simulink model "CostasLoop"  (R2025a)
settings: Solver=ode45  StartTime=0.0  StopTime=5000  RelTol=1e-3  EnableMultiTasking=on
PreLoadFcn:
  | CostasLoop_PreLoadFcn
undefined symbols (not defined in the file): h, k_i, k_p, S, vsva2197, xcvc1902
libraries: hdlBasic x33, dspmlti4 x2, hdlUtilities x1, vmcUtilities x1
settings Model: ExtModeTrigMode=oneshot  ExtModeArmWhenConnect=off  Creator=alexc  LastModifiedBy=robg
settings SolverCC: AlgebraicLoopSolver=TrustRegion
settings DataIOCC: SaveFormat=Array  SignalLoggingSaveFormat=ModelDataLogs  ReturnWorkspaceOutputs=off  SignalLoggingName=sigsOut
settings OptimizationCC: BlockReduction=off  BooleanDataType=off  DefaultParameterBehavior=Inlined  ExpressionDepthLimit=2147483647.0  InitFltsAndDblsToZero=on  LifeSpan=inf
settings DebuggingCC: SaveWithParameterizedLinksMsg=none  UnderspecifiedInitializationDetection=Classic  MergeDetectMultiDrivingBlocksExec=none  SignalResolutionControl=TryResolveAllWithWarning  MultiTaskDSMMsg=warning  MultiTaskCondExecSysMsg=none  FcnCallInpInsideContextMsg=warning  UnconnectedInputMsg=warning  UnconnectedOutputMsg=warning  UnconnectedLineMsg=warning  StateNameClashWarn=warning  SFUnexpectedBacktrackingDiag=warning  SFNoUnconditionalDefaultTransitionDiag=warning  SFExecutionAtInitializationDiag=none  ArithmeticOperatorsInVariantConditions=warning
settings HardwareCC: ProdBitPerPointer=32.0  ProdBitPerSizeT=32.0  ProdBitPerPtrDiffT=32.0  ProdLargestAtomicFloat=None  ProdIntDivRoundTo=Undefined  ProdEndianess=Unspecified  ProdWordSize=32.0  ProdHWDeviceType=32-bit Generic  TargetUnknown=on
settings ModelReferenceCC: EnableRefExpFcnMdlSchedulingChecks=on  PropagateSignalLabelsOutOfModel=off
settings SFSimCC: SimUseLocalCustomCode=off  CustomCodeUndefinedFunction=UseInterfaceOnly
settings RTWCC: RTWUseLocalCustomCode=off  GPUComputeCapability=3.5  DLArmComputeVersion=19.05
settings CodeAppCC: StateflowObjectComments=on
settings GRTTargetCC: TargetFcnLib=ansi_tfl_tmw.mat  TargetLangStandard=C89/C90 (ANSI)  CombineOutputUpdateFcns=off  GRTInterface=on
settings ConfigComp: CovMetricSettings=dw  CovSaveCumulativeToWorkspaceVar=on  CovSaveSingleToWorkspaceVar=on  CovExternalEMLEnable=off

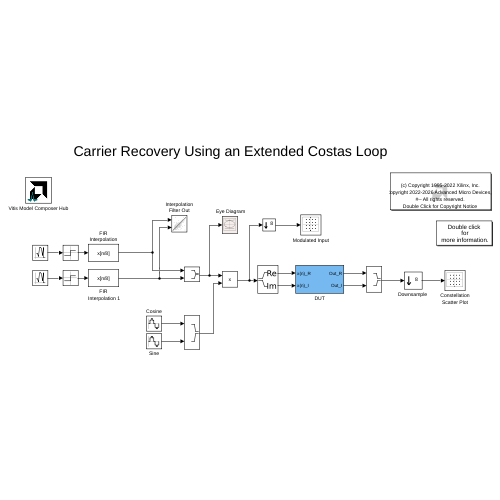
[thumbnail: Simulink's stored preview of the top-level diagram]
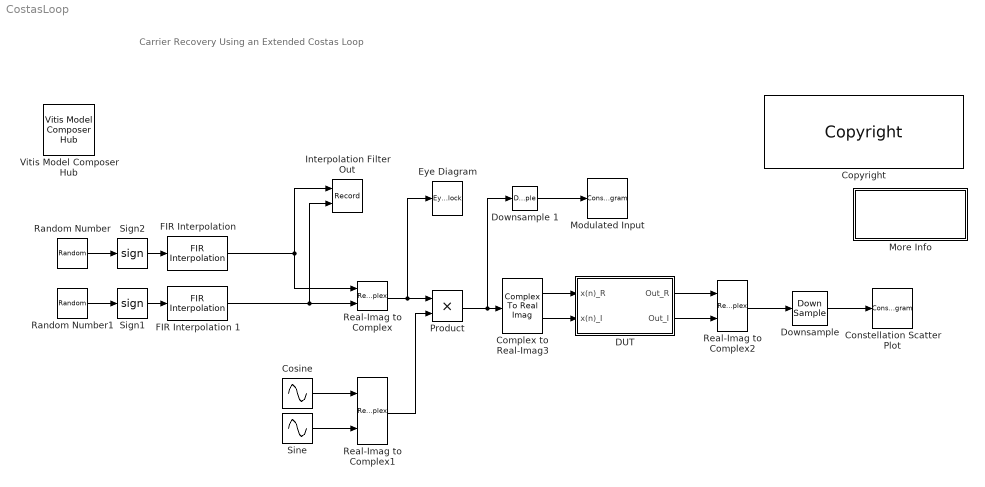
== system CostasLoop ==
  note: Carrier Recovery Using an Extended Costas Loop
  " Eye Diagram" : EyeDiagramBlock  Tag=EyeDiagram  WindowPosition=[560.000000,350.000000,800.000000,500.000000,]  Visible=on  ScopeFrameLocation=window  SamplesPerSymbol=32  SampleOffset=16  SymbolsPerTrace=1  Title=Eye Diagram  YLimits=[-2.0252 2.0024]  ColorFading=on
  Complex to Real-Imag3 : ComplexToRealImag
  Constellation Scatter Plot : ConstellationDiagram  Tag=ScatterPlot  WindowPosition=[1252.000000,116.000000,568.000000,545.000000,]  Visible=on  ScopeFrameLocation=window  SamplesPerSymbol=4  SymbolsToDisplaySource=Property  SymbolsToDisplay=40  Title=Scatter Plot  AxesLimits=[-1.5 1.5]  ColorFading=on  DefaultConfigurationName=comm.scopes.ConstellationDiagramBlockCfg
  Copyright : hdlUtilities/Copyright  copyrighttext="(c) Copyright 1995-2022 Xilinx, Inc. <br>(c) Copyright 2022-2026 Advanced Micro Devices, Inc. All rights reserved.<br><br>This document  contains proprietary, confidential information that may be used, copied and/or disclosed only as authorized by a valid licensing agreement with Advanced Micro Devices, Inc. This copyright notice must be retained on all authorized copies.<br><br> This code is provided \"as is\". Advanced Micro Devices, Inc. makes, and the end user receives, no warranties or conditions, express, implied, statutory or otherwise, and Advanced Micro Devices, Inc. specifically disclaims any implied warranties of merchantability, <br>non-infringement, or fitness for a particular purpose."  block_type=copyright
  Cosine : Sin  Frequency=2*pi*0.001/8  Phase=pi/2  SampleTime=8
  DUT : Subsystem
  "Downsample " : DownSample  N=8  InputProcessing=Inherited (this choice will be removed - see release notes)  RateOptions=Allow multirate processing
  Downsample 1 : DownSample  N=8  phase=2  InputProcessing=Inherited (this choice will be removed - see release notes)  RateOptions=Allow multirate processing
  "FIR Interpolation " : dspmlti4/FIR Interpolation  FilterSource=Dialog parameters  PrivateCoeffs=0  h=[h]  L=8  FilterObject=Hm_firinterp  InputProcessing=Columns as channels (frame based)  framing=Allow multirate processing  outputBufInitCond=0  roundingMode=Floor  overflowMode=off  firstCoeffDataTypeStr=Inherit: Same word length as input  firstCoeffMin=[]  firstCoeffMax=[]  firstCoeffLastDataTypeStr=Inherit: Same word length as input  outputDataTypeStr=Inherit: Same as accumulator  outputMin=[]  outputMax=[]  outputLastDataTypeStr=Inherit: Same as accumulator
  FIR Interpolation 1 : dspmlti4/FIR Interpolation  FilterSource=Dialog parameters  PrivateCoeffs=0  h=[h]  L=8  FilterObject=Hm_firinterp  InputProcessing=Columns as channels (frame based)  framing=Allow multirate processing  outputBufInitCond=0  roundingMode=Floor  overflowMode=off  firstCoeffDataTypeStr=Inherit: Same word length as input  firstCoeffMin=[]  firstCoeffMax=[]  firstCoeffLastDataTypeStr=Inherit: Same word length as input  outputDataTypeStr=Inherit: Same as accumulator  outputMin=[]  outputMax=[]  outputLastDataTypeStr=Inherit: Same as accumulator
  Interpolation Filter Out : Record  NumPorts=2.0  FileSettingsInternal="{\"entries\":[{\"content\":{\"excelSettings\":{\"content\":{},\"type\":\"Streamout.ExcelSettings\"},\"parquetSettings\":{\"content\":{},\"type\":\"Streamout.ParquetSettings\"}},\"type\":\"Streamout.FileSettingStorage\",\"uuid\":\"\"}],\"packageUris\":[\"http:\\/\\/schema.mathworks.com\\/mf0\\/streamout_blocks\\/R2020a\"],\"version\":\"1.0\"}"  FrameSettings=[0, 0]  Layout=[1 1]  SignalsInternal="{\"entries\":[{\"content\":{\"signals\":[{\"content\":{\"blockPath\":[],\"dimensions\":[1],\"domain\":\"\",\"lineColor\":\"#a2142f\",\"plots\":[ 1 ],\"port\":1,\"signalID\":1,\"signalName\":\"XY Graph:1\"},\"type\":\"RecordBlkView.Signal\",\"uuid\":\"\"},{\"content\":{\"blockPath\":[],\"dimensions\":[1],\"domain\":\"\",\"lineColor\":\"#139fff\",\"plots\":[ 1 ],\"port\":2,\"signalID\":2,\"signalName\":\"XY Graph:2\"},\"type\":\"RecordBlkView.Signal\",\"uuid\":\"\"}]},\"type\":\"RecordBlkView.InputSignals\",\"uuid\":\"\"}],\"packageUris\":[\"http:\\/\\/schema.mathworks.com\\/mf0\\/streamout_blocks\\/R2020a\"],\"version\":\"1.0\"}"  VisualizationBindings="{\"xyplotplugin\":{\"info\":[{\"series\":[{\"bindingParametersList\":[{\"parameter\":\"X-Axis\",\"signalID\":1,\"signalName\":\"XY Graph:1\"},{\"parameter\":\"Y-Axis\",\"signalID\":2,\"signalName\":\"XY Graph:2\"}],\"seriesID\":0}],\"subplotID\":1}]}}"  CompatibilityTag=XY  st=-1
  Modulated Input : ConstellationDiagram  Tag=ScatterPlot  WindowPosition=[37.000000,72.000000,578.000000,549.000000,]  Visible=on  ScopeFrameLocation=window  SamplesPerSymbol=4  SymbolsToDisplaySource=Property  SymbolsToDisplay=40  Title=Scatter Plot  AxesLimits=[-1.5 1.5]  ShowReferenceConstellation=off  ColorFading=on  DefaultConfigurationName=comm.scopes.ConstellationDiagramBlockCfg
  More Info : Subsystem
      mask Display: disp('Double click\n for\n more information.')
  Product : Product  InputSameDT=on  SaturateOnIntegerOverflow=on  OutDataTypeStr=Inherit: Same as first input
  Random Number : RandomNumber  SampleTime=8
  Random Number1 : RandomNumber  Seed=2  SampleTime=8
  Real-Imag to Complex : RealImagToComplex
  Real-Imag to Complex1 : RealImagToComplex
  Real-Imag to Complex2 : RealImagToComplex
  Sign1 : Signum
  Sign2 : Signum
  Sine : Sin  Frequency=2*pi*0.001/8  SampleTime=8
  Vitis Model Composer Hub : vmcUtilities/Vitis Model Composer Hub  Tag=genX  CodeGeneration=off  SubsystemName=DUT  BlockHierPath=CostasLoop/DUT  CompilationType=HDLCompilation  SubsystemType=HDLNode  ExportTypeV2=IP Catalog  StartColumn=1  NumberOfColumns=1  TargetDirectory=./netlist  exportDesign=on  analyzeDesign=off  validateDesignOnHw=off  ExportType=System Generator  IpVendor=xilinx.com  IpLibrary=hls  IpVersion=1.0  IpHWLanguage=Verilog  AieCompilerOptions={}  AieSimulatorOptions={}  CreateTestbench=off  TestbenchStackSize=10  RunRtlSim=off  RunCSim=off  RunAieSim=off  enableSimulationTimeout=on  enableGraphIterations=on  AieSimTimeout=50000  AieGraphIterations=-1  RunAieSimProfiling=off  LaunchVitisAnalyzer=off  PlotOutput=off  RunX86Sim=off  X86SimTimeout=10  GenHwImage=off  GenLibadfXo=off  GenHwValidationCode=off  PlatformType=Not Specified  HwSystemType=Baremetal  HwValidationTarget=hw  ProjDevice=xcvc1902-vsva2197-1LP-e-S  ProjDevicePart=xcvc1902-vsva2197-1LP-e-S  AIEType=AIE  SamplePeriod=-1  ClockFrequency=200  DataPathParallelism=1  xilinxfamily=versalaicore  part=xcvc1902  speed=-1LP-e-S  package=vsva2197  directory=./netlist/ip/DUT/src  testbench=off  incr_netlist=off  synthesis_tool=Vivado  clock_wrapper=Clock Enables  dbl_ovrd=According to Block Masks  dcm_input_clock_period=10  sysclk_period=10  simulink_period=1  eval_field=0  IPInfoJsonString="{\"DUTSubsystemName\":\"DUT\",\"HDLSubsystem\":{\"SubsystemName\":\"DUT\",\"IPName\":\"DUT\",\"IPLibrary\":\"VMC\",\"IPVendor\":\"User Company\",\"IPVersion\":\"1.0\",\"TargetDirectory\":\"./netlist\",\"SubsystemDir\":\"./netlist/ip/DUT\",\"FreqHz\":\"100000000\"},\"SubsystemTag\":\"HDLNode\"}"  LogFileName=/proj/xhdhdstaff5/sdegala/Head1/HEAD/ModelComposer_Sept16/Vitis_Model_Composer/Examples/HDL/Digital_Communications/Costas_loop_carrier_recovery/netlist/model_composer.log  NThreads=4  IPConfigFile=/tmp/vmctmp-9769773316677438567/CostasLoop_ipconfig.json
  wires:
  Sign1/1 -> FIR Interpolation 1/1
  Sign2/1 -> "FIR Interpolation "/1
  Real-Imag to Complex/1 -> Product/1, " Eye Diagram"/1
  Product/1 -> Complex to Real-Imag3/1, Downsample 1/1
  DUT/1(Out_R) -> Real-Imag to Complex2/1
  DUT/2(Out_I) -> Real-Imag to Complex2/2
  Real-Imag to Complex1/1 -> Product/2
  Cosine/1 -> Real-Imag to Complex1/1
  Downsample 1/1 -> Modulated Input/1
  Random Number/1 -> Sign2/1
  Random Number1/1 -> Sign1/1
  Complex to Real-Imag3/1 -> DUT/1(x(n)_R)
  Complex to Real-Imag3/2 -> DUT/2(x(n)_I)
  Real-Imag to Complex2/1 -> "Downsample "/1
  Sine/1 -> Real-Imag to Complex1/2
  "FIR Interpolation "/1 -> Interpolation Filter Out/1, Real-Imag to Complex/1
  FIR Interpolation 1/1 -> Real-Imag to Complex/2, Interpolation Filter Out/2
  "Downsample "/1 -> Constellation Scatter Plot/1

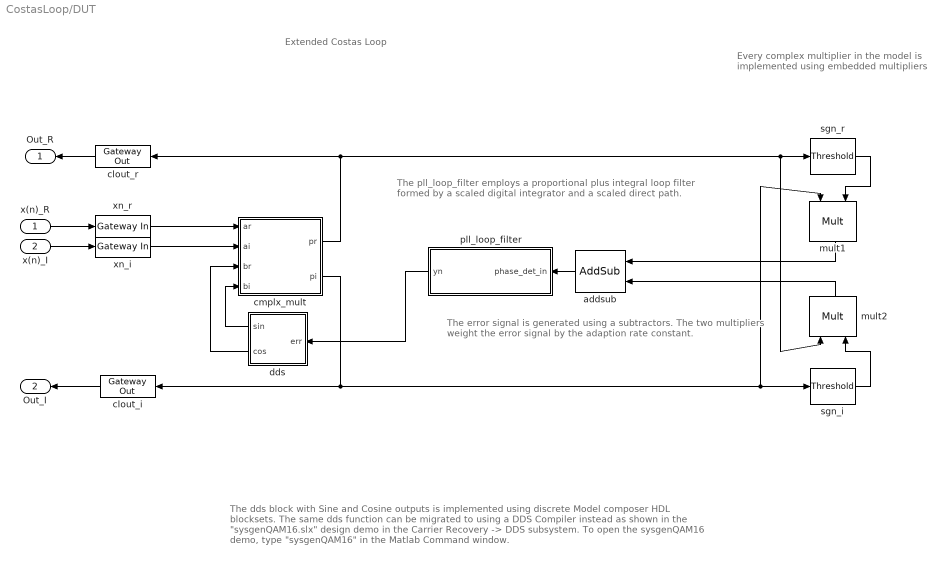
== system CostasLoop/DUT ==
  note: Extended Costas Loop
  note: The error signal is generated using a subtractors.  The
      | two multipliers weight  the error signal by the adaption
      | rate constant.
  note: The pll_loop_filter employs a proportional plus integral
      | loop filter formed by a scaled digital integrator
      | and a scaled direct path.
  note: Every complex multiplier in the model is
      | implemented using embedded multipliers
  note: The dds block with Sine and Cosine outputs is implemented using discrete Model composer HDL blocksets.
      | The same dds function can be migrated to using a DDS Compiler instead as shown in the "sysgenQAM16.slx"
      | design demo in the Carrier Recovery -> DDS subsystem. To open the sysgenQAM16 demo, type "sysgenQAM16"
      | in the Matlab Command window.
  x(n)_R : Inport
  x(n)_I : Inport  Port=2
  addsub : hdlBasic/AddSub  mode=Subtraction  use_carryin=off  use_carryout=off  en=off  latency=0  precision=User Defined  arith_type="Signed  (2's comp)"  n_bits=16  bin_pt=13  quantization="Round  (unbiased: +/- Inf)"  overflow=Saturate  use_behavioral_HDL=on  hw_selection=Fabric  pipelined=off  use_rpm=off  XmcBlockStatus=1  maskContainerNames=tabcontainer1  block_type=addsub  block_config=sysgen:Addsub_config
  clout_i : hdlBasic/Gateway Out  inherit_from_input=off  bool_to_boolean=off  hdl_port=on  rows=1  columns=1  UseAsDAC=off  DACChannel='1'  interface=None  automatic_assignment=on  address_offset=hex2dec('00')  intf_name=''  intf_description=''  timing_constraint=None  locs_specified=off  LOCs={}  io_standard={}  XmcBlockStatus=1  maskContainerNames=group4  block_type=gatewayout  block_config=sysgen:gateway_out_config  block_width_w=590  block_height_w=620  block_width=620  block_height=750
  clout_r : hdlBasic/Gateway Out  inherit_from_input=off  bool_to_boolean=off  hdl_port=on  rows=1  columns=1  UseAsDAC=off  DACChannel='1'  interface=None  automatic_assignment=on  address_offset=hex2dec('00')  intf_name=''  intf_description=''  timing_constraint=None  locs_specified=off  LOCs={}  io_standard={}  XmcBlockStatus=1  maskContainerNames=group4  block_type=gatewayout  block_config=sysgen:gateway_out_config  block_width_w=590  block_height_w=620  block_width=620  block_height=750
  cmplx_mult : Subsystem
  dds : Subsystem
  mult1 : hdlBasic/Mult  precision=User Defined  arith_type="Signed  (2's comp)"  n_bits=16  bin_pt=13  quantization="Round  (unbiased: +/- Inf)"  overflow=Wrap  en=off  latency=0  opt_float=off  fp_mult_usage=No Usage  use_behavioral_HDL=off  opt=Speed  use_embedded=on  optimum_pipeline=off  pipeline=off  use_rpm=off  placement_style=Rectangular shape  XmcBlockStatus=1  maskContainerNames=group1  block_type=mult  block_config=sysgen:Mult_config  block_width=598  block_height=876
  mult2 : hdlBasic/Mult  precision=User Defined  arith_type="Signed  (2's comp)"  n_bits=16  bin_pt=13  quantization="Round  (unbiased: +/- Inf)"  overflow=Wrap  en=off  latency=0  opt_float=off  fp_mult_usage=No Usage  use_behavioral_HDL=off  opt=Speed  use_embedded=on  optimum_pipeline=off  pipeline=off  use_rpm=off  placement_style=Rectangular shape  XmcBlockStatus=1  maskContainerNames=group1  block_type=mult  block_config=sysgen:Mult_config  block_width=598  block_height=876
  pll_loop_filter : Subsystem
  sgn_i : hdlBasic/Threshold  en=off  latency=0  XmcBlockStatus=1  maskContainerNames=group2  block_type=sgn  block_config=sysgen:Sgn_config
  sgn_r : hdlBasic/Threshold  en=off  latency=0  XmcBlockStatus=1  maskContainerNames=group2  block_type=sgn  block_config=sysgen:Sgn_config
  xn_i : hdlBasic/Gateway In  gui_display_data_type=Fixed-point  arith_type=Signed (2's comp)  n_bits=8  bin_pt=6  preci_type=Single  exp_width=8  frac_width=24  rows=1  columns=1  quantization="Round  (unbiased: +/- Inf)"  overflow=Saturate  period=1  UseAsADC=off  ADCChannel='1'  interface=None  automatic_assignment=on  address_offset=hex2dec('00')  intf_name=''  intf_description=''  default_value=0  timing_constraint=None  locs_specified=off  LOCs={}  io_standard={}  inherit_from_input=off  hdl_port=on  XmcBlockStatus=1  maskContainerNames=group4  block_type=gatewayin  block_config=sysgen:gateway_in_config  block_width_w=590  block_height_w=620  block_width=640  block_height=850
  xn_r : hdlBasic/Gateway In  gui_display_data_type=Fixed-point  arith_type=Signed (2's comp)  n_bits=8  bin_pt=6  preci_type=Single  exp_width=8  frac_width=24  rows=1  columns=1  quantization="Round  (unbiased: +/- Inf)"  overflow=Saturate  period=1  UseAsADC=off  ADCChannel='1'  interface=None  automatic_assignment=on  address_offset=hex2dec('00')  intf_name=''  intf_description=''  default_value=0  timing_constraint=None  locs_specified=off  LOCs={}  io_standard={}  inherit_from_input=off  hdl_port=on  XmcBlockStatus=1  maskContainerNames=group4  block_type=gatewayin  block_config=sysgen:gateway_in_config  block_width_w=590  block_height_w=620  block_width=640  block_height=850
  Out_R : Outport
  Out_I : Outport  Port=2
  wires:
  clout_r/1 -> Out_R/1
  cmplx_mult/1(pr) -> mult2/1, sgn_r/1, clout_r/1
  mult2/1 -> addsub/2
  mult1/1 -> addsub/1
  addsub/1 -> pll_loop_filter/1(phase_det_in)
  sgn_r/1 -> mult1/2
  sgn_i/1 -> mult2/2
  dds/1(sin) -> cmplx_mult/4(bi)
  pll_loop_filter/1(yn) -> dds/1(err)
  clout_i/1 -> Out_I/1
  cmplx_mult/2(pi) -> clout_i/1, mult1/1, sgn_i/1
  dds/2(cos) -> cmplx_mult/3(br)
  x(n)_I/1 -> xn_i/1
  xn_i/1 -> cmplx_mult/2(ai)
  x(n)_R/1 -> xn_r/1
  xn_r/1 -> cmplx_mult/1(ar)

== system CostasLoop/More Info ==
  note: This design shows an implementation of Costas Loop used for Carrier Recovery.
      | The modulated input is modeled using simulink blocks while the costas loop
      | algorithm is implemented using System Generator for DSP blocks.
      |
      | The dds block with Sine and Cosine outputs is implemented using basic
      | System Generator Blocks.The pll_loop_filter employs a proportional plus integral
      | loop filter formed by a scaled digital integrator and a scaled direct path. The error
      | signal is generated using a subtractors.  Two multipliers weight  the error signal
      | by the adaption rate constant.
      |
      |
      | For additional information on Costas Loop:
      |
      | Simon Haykin,  "Communication Systems", 4th Edition, pp. 453-454.
  note: Carrier Recovery Using an Extended Costas Loop

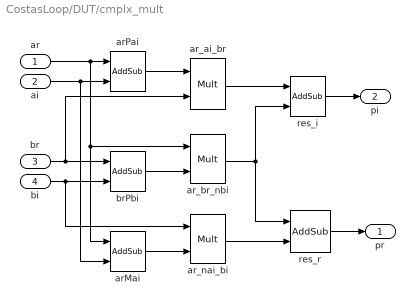
== system CostasLoop/DUT/cmplx_mult ==
  ar : Inport
  ai : Inport  Port=2
  br : Inport  Port=3
  bi : Inport  Port=4
  arMai : hdlBasic/AddSub  mode=Subtraction  use_carryin=off  use_carryout=off  en=off  latency=0  precision=User Defined  arith_type="Signed  (2's comp)"  n_bits=17  bin_pt=13  quantization="Round  (unbiased: +/- Inf)"  overflow=Saturate  use_behavioral_HDL=on  hw_selection=Fabric  pipelined=off  use_rpm=off  XmcBlockStatus=1  maskContainerNames=tabcontainer1  block_type=addsub  block_config=sysgen:Addsub_config
  arPai : hdlBasic/AddSub  mode=Addition  use_carryin=off  use_carryout=off  en=off  latency=0  precision=Full  arith_type="Signed  (2's comp)"  n_bits=17  bin_pt=13  quantization="Round  (unbiased: +/- Inf)"  overflow=Saturate  use_behavioral_HDL=on  hw_selection=Fabric  pipelined=off  use_rpm=off  XmcBlockStatus=1  maskContainerNames=tabcontainer1  block_type=addsub  block_config=sysgen:Addsub_config
  ar_ai_br : hdlBasic/Mult  precision=User Defined  arith_type="Signed  (2's comp)"  n_bits=16  bin_pt=13  quantization="Round  (unbiased: +/- Inf)"  overflow=Saturate  en=off  latency=0  opt_float=off  fp_mult_usage=No Usage  use_behavioral_HDL=off  opt=Speed  use_embedded=on  optimum_pipeline=off  pipeline=off  use_rpm=off  placement_style=Rectangular shape  XmcBlockStatus=1  maskContainerNames=group1  block_type=mult  block_config=sysgen:Mult_config  block_width=598  block_height=876
  ar_br_nbi : hdlBasic/Mult  precision=User Defined  arith_type="Signed  (2's comp)"  n_bits=16  bin_pt=13  quantization="Round  (unbiased: +/- Inf)"  overflow=Saturate  en=off  latency=0  opt_float=off  fp_mult_usage=No Usage  use_behavioral_HDL=off  opt=Speed  use_embedded=on  optimum_pipeline=off  pipeline=off  use_rpm=off  placement_style=Rectangular shape  XmcBlockStatus=1  maskContainerNames=group1  block_type=mult  block_config=sysgen:Mult_config  block_width=598  block_height=876
  ar_nai_bi : hdlBasic/Mult  precision=User Defined  arith_type="Signed  (2's comp)"  n_bits=16  bin_pt=13  quantization="Round  (unbiased: +/- Inf)"  overflow=Saturate  en=off  latency=0  opt_float=off  fp_mult_usage=No Usage  use_behavioral_HDL=off  opt=Speed  use_embedded=on  optimum_pipeline=off  pipeline=off  use_rpm=off  placement_style=Rectangular shape  XmcBlockStatus=1  maskContainerNames=group1  block_type=mult  block_config=sysgen:Mult_config  block_width=598  block_height=876
  brPbi : hdlBasic/AddSub  mode=Subtraction  use_carryin=off  use_carryout=off  en=off  latency=0  precision=Full  arith_type="Signed  (2's comp)"  n_bits=17  bin_pt=13  quantization="Round  (unbiased: +/- Inf)"  overflow=Saturate  use_behavioral_HDL=on  hw_selection=Fabric  pipelined=off  use_rpm=off  XmcBlockStatus=1  maskContainerNames=tabcontainer1  block_type=addsub  block_config=sysgen:Addsub_config
  res_i : hdlBasic/AddSub  mode=Subtraction  use_carryin=off  use_carryout=off  en=off  latency=0  precision=User Defined  arith_type="Signed  (2's comp)"  n_bits=17  bin_pt=13  quantization="Round  (unbiased: +/- Inf)"  overflow=Saturate  use_behavioral_HDL=on  hw_selection=Fabric  pipelined=off  use_rpm=off  XmcBlockStatus=1  maskContainerNames=tabcontainer1  block_type=addsub  block_config=sysgen:Addsub_config
  res_r : hdlBasic/AddSub  mode=Addition  use_carryin=off  use_carryout=off  en=off  latency=0  precision=User Defined  arith_type="Signed  (2's comp)"  n_bits=17  bin_pt=13  quantization="Round  (unbiased: +/- Inf)"  overflow=Saturate  use_behavioral_HDL=on  hw_selection=Fabric  pipelined=off  use_rpm=off  XmcBlockStatus=1  maskContainerNames=tabcontainer1  block_type=addsub  block_config=sysgen:Addsub_config
  pr : Outport
  pi : Outport  Port=2
  wires:
  res_r/1 -> pr/1
  ar_nai_bi/1 -> res_r/2
  arMai/1 -> ar_nai_bi/2
  res_i/1 -> pi/1
  ar_ai_br/1 -> res_i/1
  ar_br_nbi/1 -> res_r/1, res_i/2
  brPbi/1 -> ar_br_nbi/2
  arPai/1 -> ar_ai_br/1
  bi/1 -> ar_nai_bi/1, brPbi/2
  br/1 -> ar_ai_br/2, brPbi/1
  ai/1 -> arMai/2, arPai/2
  ar/1 -> ar_br_nbi/1, arMai/1, arPai/1

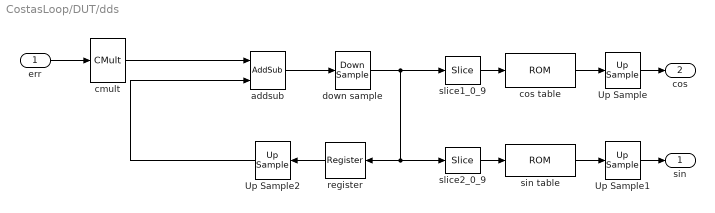
== system CostasLoop/DUT/dds ==
  err : Inport
  Up Sample : hdlBasic/Up Sample  sample_ratio=64  copy_samples=on  en=off  latency=0  XmcBlockStatus=1  maskContainerNames=group1  block_type=usamp  block_config=sysgen:Upsample_config
  Up Sample1 : hdlBasic/Up Sample  sample_ratio=64  copy_samples=on  en=off  latency=0  XmcBlockStatus=1  maskContainerNames=group1  block_type=usamp  block_config=sysgen:Upsample_config
  Up Sample2 : hdlBasic/Up Sample  sample_ratio=64  copy_samples=on  en=off  latency=0  XmcBlockStatus=1  maskContainerNames=group1  block_type=usamp  block_config=sysgen:Upsample_config
  addsub : hdlBasic/AddSub  mode=Addition  use_carryin=off  use_carryout=off  en=off  latency=0  precision=User Defined  arith_type="Signed  (2's comp)"  n_bits=32  bin_pt=0  quantization="Round  (unbiased: +/- Inf)"  overflow=Wrap  use_behavioral_HDL=on  hw_selection=Fabric  pipelined=off  use_rpm=off  XmcBlockStatus=1  maskContainerNames=tabcontainer1  block_type=addsub  block_config=sysgen:Addsub_config
  cmult : hdlBasic/CMult  const=1024  gui_display_data_type=Fixed-point  const_n_bits=16  const_bin_pt=0  float_type=Single  exp_bits=8  fraction_bits=24  en=off  latency=0  precision=User Defined  arith_type="Signed  (2's comp)"  n_bits=32  bin_pt=0  quantization=Truncate  overflow=Wrap  use_behavioral_HDL=off  mem_type=Distributed RAM  pipeline=off  use_rpm=off  placement_style=Rectangular Shape  XmcBlockStatus=1  maskContainerNames=tabcontainer1  block_type=cmult  block_config=sysgen:CMult_config
      settings: infoedit=[]
  cos table : hdlBasic/ROM  depth=1024  initVector=cos([0:1023]*2*pi/1024)  distributed_mem=Block RAM  rst=off  init_reg=0  en=off  latency=1  gui_display_data_type=Fixed-point  arith_type="Signed  (2's comp)"  n_bits=8  bin_pt=6  preci_type=Single  exp_width=8  frac_width=24  optimize=Area  use_rpm=off  simulation_type=fast_sim  XmcBlockStatus=1  maskContainerNames=tabcontainer1  block_type=sprom  block_config=sysgen:SPROM_config
  down sample : hdlBasic/Down Sample  sample_ratio=64  sample_phase=First Value of Frame  en=off  rst=off  latency=0  XmcBlockStatus=1  maskContainerNames=group1  block_type=dsamp  block_config=sysgen:Downsample_config
  register : hdlBasic/Register  init=0  rst=off  en=off  XmcBlockStatus=1  maskContainerNames=tabcontainer1  block_type=register  block_config=sysgen:Register_config
  sin table : hdlBasic/ROM  depth=1024  initVector=-sin([0:1023]*2*pi/1024)  distributed_mem=Block RAM  rst=off  init_reg=0  en=off  latency=1  gui_display_data_type=Fixed-point  arith_type="Signed  (2's comp)"  n_bits=8  bin_pt=6  preci_type=Single  exp_width=8  frac_width=24  optimize=Area  use_rpm=off  simulation_type=fast_sim  XmcBlockStatus=1  maskContainerNames=tabcontainer1  block_type=sprom  block_config=sysgen:SPROM_config
  slice1_0_9 : hdlBasic/Slice  nbits=10  boolean_output=off  mode=Lower Bit Location + Width  bit1=0  base1=MSB of Input  bit0=0  base0=LSB of Input  XmcBlockStatus=1  maskContainerNames=group1  block_type=slice  block_config=sysgen:Slice_config
  slice2_0_9 : hdlBasic/Slice  nbits=10  boolean_output=off  mode=Lower Bit Location + Width  bit1=0  base1=MSB of Input  bit0=0  base0=LSB of Input  XmcBlockStatus=1  maskContainerNames=group1  block_type=slice  block_config=sysgen:Slice_config
  sin : Outport
  cos : Outport  Port=2
  wires:
  err/1 -> cmult/1
  cmult/1 -> addsub/1
  addsub/1 -> down sample/1
  down sample/1 -> slice1_0_9/1, slice2_0_9/1, register/1
  slice1_0_9/1 -> cos table/1
  slice2_0_9/1 -> sin table/1
  cos table/1 -> Up Sample/1
  Up Sample/1 -> cos/1
  sin table/1 -> Up Sample1/1
  Up Sample1/1 -> sin/1
  Up Sample2/1 -> addsub/2
  register/1 -> Up Sample2/1

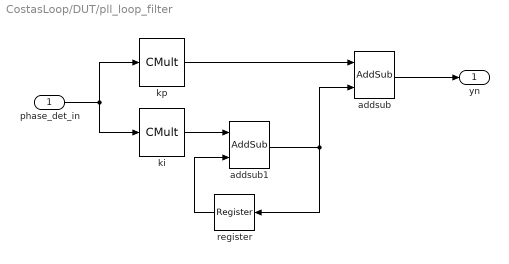
== system CostasLoop/DUT/pll_loop_filter ==
  phase_det_in : Inport
  addsub : hdlBasic/AddSub  mode=Addition  use_carryin=off  use_carryout=off  en=off  latency=0  precision=User Defined  arith_type=Unsigned  n_bits=32  bin_pt=28  quantization="Round  (unbiased: +/- Inf)"  overflow=Wrap  use_behavioral_HDL=on  hw_selection=Fabric  pipelined=off  use_rpm=off  XmcBlockStatus=1  maskContainerNames=tabcontainer1  block_type=addsub  block_config=sysgen:Addsub_config
  addsub1 : hdlBasic/AddSub  mode=Addition  use_carryin=off  use_carryout=off  en=off  latency=0  precision=User Defined  arith_type="Signed  (2's comp)"  n_bits=32  bin_pt=28  quantization="Round  (unbiased: +/- Inf)"  overflow=Wrap  use_behavioral_HDL=on  hw_selection=Fabric  pipelined=off  use_rpm=off  XmcBlockStatus=1  maskContainerNames=tabcontainer1  block_type=addsub  block_config=sysgen:Addsub_config
  ki : hdlBasic/CMult  const=k_i  gui_display_data_type=Fixed-point  const_n_bits=16  const_bin_pt=15  float_type=Single  exp_bits=8  fraction_bits=24  en=off  latency=0  precision=User Defined  arith_type="Signed  (2's comp)"  n_bits=32  bin_pt=28  quantization="Round  (unbiased: +/- Inf)"  overflow=Wrap  use_behavioral_HDL=off  mem_type=Distributed RAM  pipeline=off  use_rpm=off  placement_style=Rectangular Shape  XmcBlockStatus=1  maskContainerNames=tabcontainer1  block_type=cmult  block_config=sysgen:CMult_config
      settings: infoedit=[]
  kp : hdlBasic/CMult  const=k_p  gui_display_data_type=Fixed-point  const_n_bits=16  const_bin_pt=15  float_type=Single  exp_bits=8  fraction_bits=24  en=off  latency=0  precision=User Defined  arith_type="Signed  (2's comp)"  n_bits=32  bin_pt=28  quantization="Round  (unbiased: +/- Inf)"  overflow=Wrap  use_behavioral_HDL=off  mem_type=Distributed RAM  pipeline=off  use_rpm=off  placement_style=Rectangular Shape  XmcBlockStatus=1  maskContainerNames=tabcontainer1  block_type=cmult  block_config=sysgen:CMult_config
      settings: infoedit=[]
  register : hdlBasic/Register  init=0  rst=off  en=off  XmcBlockStatus=1  maskContainerNames=tabcontainer1  block_type=register  block_config=sysgen:Register_config
  yn : Outport
  wires:
  ki/1 -> addsub1/1
  phase_det_in/1 -> ki/1, kp/1
  register/1 -> addsub1/2
  addsub1/1 -> addsub/2, register/1
  kp/1 -> addsub/1
  addsub/1 -> yn/1
